simulink model "RRpendulum_digtwin_BLDC"  (R2024b)
settings: Solver=FixedStepAuto  StartTime=0.0  StopTime=inf  FixedStep=0.001  RelTol=1e-3  EnableMultiTasking=on
PreLoadFcn:
  | %define mechanical pars, init conditions
  | run RRpendulum_kinctrl_numericalsetup.mlx
  | 
  | %% parameters moved to model workspace
  | % sample time
  | %T_SAMPLE = 0.001;
  | 
  | %microsteps per turn of 200 step motor @ x16 microstepping
  | %STEPS_PER_TURN = 3200;
  | 
  | %encoder counts per turn
  | %COUNTS_PER_TURN = 2400;
model workspace (MAT data in the model file):
  COUNTS_PER_TURN_MOT = 8192
  COUNTS_PER_TURN_PEND = 2400
  MOTOR_VEL_RESOLUTION_DIV = 4
  PEND_VEL_RESOLUTION_DIV = 1
  T_SAMPLE = 0.001
undefined symbols (not defined in the file): b1_num, b2_num, dspblkCoreblockFVToolHelper, g_num, gcbh, l_num, m_num, q1_0, q2_0, r_num, satlimits, T01_num0, T12_num0, v1_0, v2_0, X, Y, Z
libraries: sm_lib x12, nesl_utility x7, simulink x2, fl_lib x2, ee_lib x2, raspberrypiCommlib x1
(part 2 of 2)

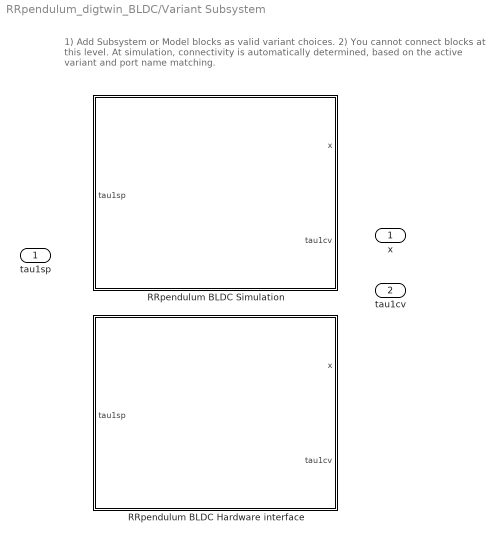
== system RRpendulum_digtwin_BLDC/Variant Subsystem ==
  note: 1) Add Subsystem or Model blocks as valid variant choices.
      | 2) You cannot connect blocks at this level. At simulation, connectivity is automatically
      | determined, based on the active variant and port name matching.
  tau1sp : Inport
  RRpendulum BLDC Hardware interface : Subsystem  VariantControl=(codegen)  mask{t_sample=T_SAMPLE, enc_cpt=COUNTS_PER_TURN_PEND, mot_cpt=COUNTS_PER_TURN_MOT, Nv2filt=10}
      mask prompts: t_sample "Sample time (s)"; enc_cpt "Pendulum Encoder CPT (x4)"; mot_cpt "Motor Encoder CPT (x4)"; Nv2filt "Moving average filter"
      mask Display:
      | image('pendulum_down_physical.PNG');
      | port_label('input', 1, 'tau1sp');
      | port_label('output', 1, 'x');
      | port_label('output', 2, 'tau1cv');
  RRpendulum BLDC Simulation : Subsystem  VariantControl=(sim)  mask{initstate=[q1_0; v1_0 ;q2_0; v2_0], satlimits=satlimits, g=g_num, m=m_num, r=r_num, l=l_num, b=[b1_num b2_num]}
      mask prompts: initstate "Initial state: [q1; v1; q2; v2]"; satlimits "Saturation limits axis 1: [vdot1max;v1max]"; g "Gravity: g"; m "Mass: m"; r "Radius: r"; l "Length: l"; b "Viscous damping factors: [b1;b2]"
      mask DialogControl MechanismGroupVar Prompt: Mechanism
      mask Display:
      | image('pendulum_down_simulation.PNG');
      | port_label('input', 1, 'tau1sp');
      | port_label('output', 1, 'x');
      | port_label('output', 2, 'tau1cv');
  x : Outport
  tau1cv : Outport  Port=2

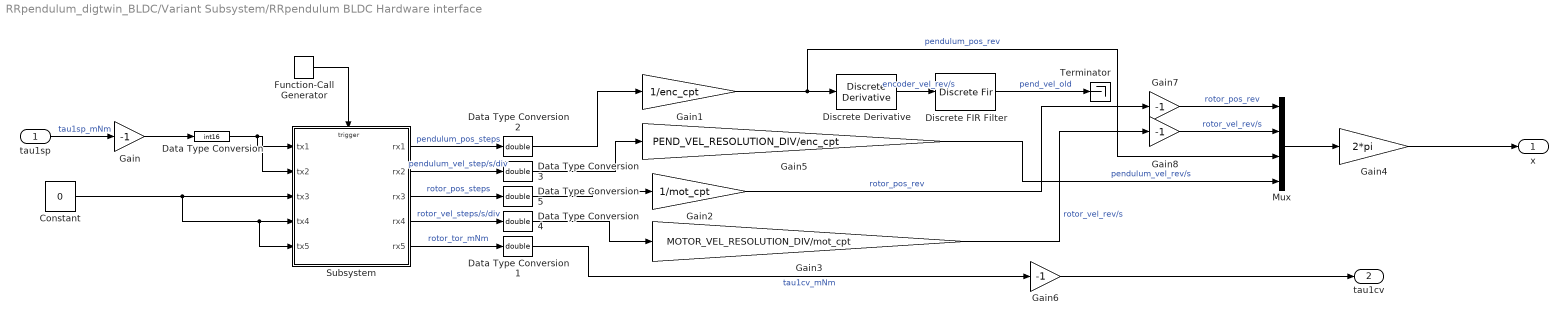
== system RRpendulum_digtwin_BLDC/Variant Subsystem/RRpendulum BLDC Hardware interface ==
  tau1sp : Inport
  Constant : Constant  Value=0  OutDataTypeStr=int16
  Data Type Conversion : DataTypeConversion  OutDataTypeStr=int16  SaturateOnIntegerOverflow=off  RndMeth=Floor
  Data Type Conversion{1..5} (5 alike) : DataTypeConversion  OutDataTypeStr=double  SaturateOnIntegerOverflow=off  RndMeth=Floor
  Discrete Derivative : simulink/Discrete/Discrete Derivative  gainval=1.0  ICPrevScaledInput=0.0  OutMin=[]  OutMax=[]  OutDataType=fixdt(1, 16)  OutScaling=2^-10  DoSatur=off
  Discrete FIR Filter : DiscreteFir  LoadFcn=dspblkCoreblockFVToolHelper(gcbh,'load');  Coefficients=ones(1,Nv2filt)/Nv2filt
      settings: CopyFcn=dspblkCoreblockFVToolHelper(gcbh,'copy');  DeleteFcn=dspblkCoreblockFVToolHelper(gcbh,'close');  ModelCloseFcn=dspblkCoreblockFVToolHelper(gcbh,'close');  PreSaveFcn=dspblkCoreblockFVToolHelper(gcbh,'presave');  PostSaveFcn=dspblkCoreblockFVToolHelper(gcbh,'postsave');  CloseFcn=dspblkCoreblockFVToolHelper(gcbh,'close');
  Function-Call Generator : simulink/Ports & Subsystems/Function-Call Generator  sample_time=t_sample  numberOfIterations=1  DisallowWideOutput=off
  Gain{,6..8} (4 alike) : Gain  Gain=-1
  Gain1 : Gain  Gain=1/enc_cpt
  Gain2 : Gain  Gain=1/mot_cpt
  Gain3 : Gain  Gain=MOTOR_VEL_RESOLUTION_DIV/mot_cpt
  Gain4 : Gain  Gain=2*pi
  Gain5 : Gain  Gain=PEND_VEL_RESOLUTION_DIV/enc_cpt
  Mux : Mux
  Subsystem : Subsystem
  Terminator : Terminator
  x : Outport
  tau1cv : Outport  Port=2
  wires:
  Data Type Conversion2/1 -> Gain1/1
  Data Type Conversion/1 -> Subsystem/2(tx2), Subsystem/1(tx1)
  Gain1/1 -> Discrete Derivative/1, Mux/3  "pendulum_pos_rev"
  Data Type Conversion3/1 -> Gain5/1
  Subsystem/1(rx1) -> Data Type Conversion2/1  "pendulum_pos_steps"
  Function-Call Generator/1 -> Subsystem/Trigger
  Subsystem/2(rx2) -> Data Type Conversion3/1  "pendulum_vel_step/s/div"
  Subsystem/4(rx4) -> Data Type Conversion4/1  "rotor_vel_steps/s/div"
  Gain3/1 -> Gain8/1  "rotor_vel_rev/s"
  Constant/1 -> Subsystem/5(tx5), Subsystem/4(tx4), Subsystem/3(tx3)
  Data Type Conversion4/1 -> Gain3/1
  tau1sp/1 -> Gain/1  "tau1sp_mNm"
  Gain2/1 -> Gain7/1  "rotor_pos_rev"
  Discrete Derivative/1 -> Discrete FIR Filter/1  "encoder_vel_rev/s"
  Mux/1 -> Gain4/1
  Discrete FIR Filter/1 -> Terminator/1  "pend_vel_old"
  Subsystem/5(rx5) -> Data Type Conversion1/1  "rotor_tor_mNm"
  Gain4/1 -> x/1
  Data Type Conversion1/1 -> Gain6/1  "tau1cv_mNm"
  Gain5/1 -> Mux/4  "pendulum_vel_rev/s"
  Subsystem/3(rx3) -> Data Type Conversion5/1  "rotor_pos_steps"
  Data Type Conversion5/1 -> Gain2/1
  Gain/1 -> Data Type Conversion/1
  Gain6/1 -> tau1cv/1
  Gain7/1 -> Mux/1  "rotor_pos_rev"
  Gain8/1 -> Mux/2  "rotor_vel_rev/s"

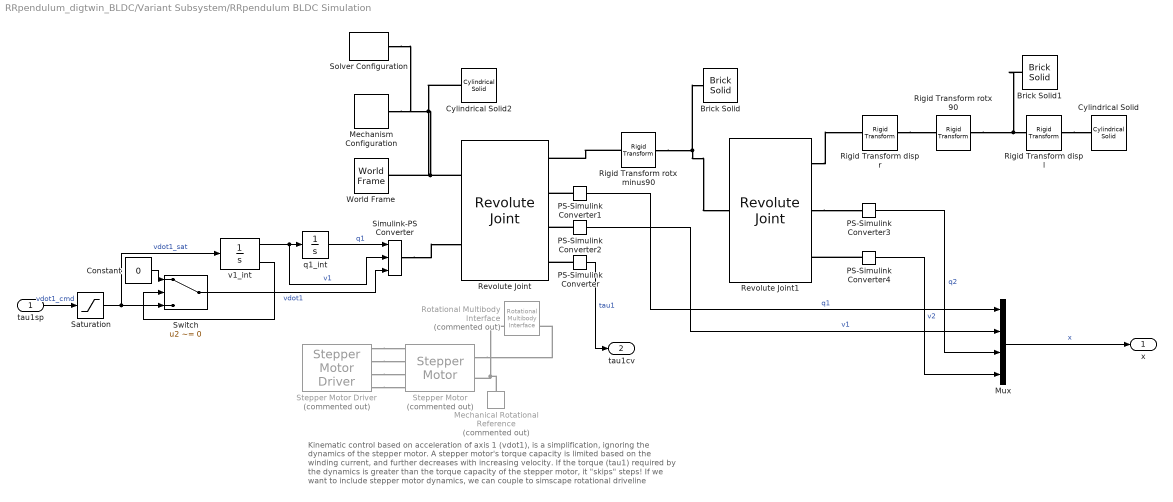
== system RRpendulum_digtwin_BLDC/Variant Subsystem/RRpendulum BLDC Simulation ==
  note: Kinematic control based on acceleration of axis 1 (vdot1), is a simplification, ignoring the dynamics of the stepper motor.
      |
      | A stepper motor's torque capacity is limited based on the winding current, and further decreases with increasing velocity. If the torque (tau1) required by the dynamics is greater than the torque capacity of the stepper motor, it "skips" steps!
      |
      | If we want to include stepper motor dynamics, we can couple to simscape rotational driveline
  tau1sp : Inport
  Brick Solid : sm_lib/Body Elements/Brick Solid  BrickDimensions=[0.001 0.001 r_num]  BrickDimensionsUnits=m  ExportEntireGeometry=off  InertiaType=CalculateFromGeometry  BasedOnType=Mass  Density=1000  DensityUnits=kg/m^3  Mass=0  MassUnits=kg  CenterOfMass=[0 0 0]  CenterOfMassUnits=m  MomentsOfInertia=[1 1 1]  MomentsOfInertiaUnits=kg*m^2  ProductsOfInertia=[0 0 0]  ProductsOfInertiaUnits=kg*m^2  GraphicType=FromGeometry  MarkerShape=Sphere  MarkerSize=10  GraphicVisPropType=SimpleVisualProperties  GraphicDiffuseColor=[0.5 0.5 0.5]  GraphicOpacity=1  GraphicSpecularColor=[0.5 0.5 0.5 1.0]  GraphicAmbientColor=[0.15 0.15 0.15 1.0]  GraphicEmissiveColor=[0.0 0.0 0.0 1.0]  GraphicShininess=75  DoExposeReferenceFrame=on  SerializedFrames=<Frames><Frame><Id>Frame1</Id><Value><Name>F1</Name><Origin><Source>GeometricFeature</Source><FeatureName>-z surface</FeatureName></Origin><PrimaryAxis><DefinedDirection>-Z</DefinedDirection><Source>GeometricFeature</Source><SourceDirection>+Z</SourceDirection><FeatureName>-z surface</FeatureName></PrimaryAxis><SecondaryAxis><DefinedDirection>+X</DefinedDirection><Source>ReferenceFrame</Source><SourceDirection>+X</SourceDirection><FeatureName></FeatureName></SecondaryAxis></Value></Frame></Frames>
  Brick Solid1 : sm_lib/Body Elements/Brick Solid  BrickDimensions=[0.001 0.001 l_num]  BrickDimensionsUnits=m  ExportEntireGeometry=off  InertiaType=CalculateFromGeometry  BasedOnType=Mass  Density=1000  DensityUnits=kg/m^3  Mass=0  MassUnits=kg  CenterOfMass=[0 0 0]  CenterOfMassUnits=m  MomentsOfInertia=[1 1 1]  MomentsOfInertiaUnits=kg*m^2  ProductsOfInertia=[0 0 0]  ProductsOfInertiaUnits=kg*m^2  GraphicType=FromGeometry  MarkerShape=Sphere  MarkerSize=10  GraphicVisPropType=SimpleVisualProperties  GraphicDiffuseColor=[0.5 0.5 0.5]  GraphicOpacity=1  GraphicSpecularColor=[0.5 0.5 0.5 1.0]  GraphicAmbientColor=[0.15 0.15 0.15 1.0]  GraphicEmissiveColor=[0.0 0.0 0.0 1.0]  GraphicShininess=75  DoExposeReferenceFrame=on  SerializedFrames=<Frames><Frame><Id>Frame1</Id><Value><Name>F1</Name><Origin><Source>GeometricFeature</Source><FeatureName>-z surface</FeatureName></Origin><PrimaryAxis><DefinedDirection>+Z</DefinedDirection><Source>GeometricFeature</Source><SourceDirection>+Z</SourceDirection><FeatureName>-z surface</FeatureName></PrimaryAxis><SecondaryAxis><DefinedDirection>+X</DefinedDirection><Source>ReferenceFrame</Source><SourceDirection>+X</SourceDirection><FeatureName></FeatureName></SecondaryAxis></Value></Frame></Frames>
  Constant : Constant  Value=0
  Cylindrical Solid : sm_lib/Body Elements/Cylindrical Solid  CylinderRadius=5  CylinderRadiusUnits=mm  CylinderLength=30  CylinderLengthUnits=mm  ExportEntireGeometry=off  InertiaType=PointMass  BasedOnType=Mass  Density=1000  DensityUnits=kg/m^3  Mass=m  MassUnits=kg  CenterOfMass=[0 0 0]  CenterOfMassUnits=m  MomentsOfInertia=[1 1 1]  MomentsOfInertiaUnits=kg*m^2  ProductsOfInertia=[0 0 0]  ProductsOfInertiaUnits=kg*m^2  GraphicType=FromGeometry  MarkerShape=Sphere  MarkerSize=10  GraphicVisPropType=SimpleVisualProperties  GraphicDiffuseColor=[0.5 0.5 0.5]  GraphicOpacity=1  GraphicSpecularColor=[0.5 0.5 0.5 1.0]  GraphicAmbientColor=[0.15 0.15 0.15 1.0]  GraphicEmissiveColor=[0.0 0.0 0.0 1.0]  GraphicShininess=75  DoExposeReferenceFrame=on  SerializedFrames=<Frames/>
  Cylindrical Solid2 : sm_lib/Body Elements/Cylindrical Solid  CylinderRadius=0.1*r_num  CylinderRadiusUnits=m  CylinderLength=l_num*1.25  CylinderLengthUnits=m  ExportEntireGeometry=off  InertiaType=CalculateFromGeometry  BasedOnType=Mass  Density=1000  DensityUnits=kg/m^3  Mass=0  MassUnits=kg  CenterOfMass=[0 0 0]  CenterOfMassUnits=m  MomentsOfInertia=[1 1 1]  MomentsOfInertiaUnits=kg*m^2  ProductsOfInertia=[0 0 0]  ProductsOfInertiaUnits=kg*m^2  GraphicType=FromGeometry  MarkerShape=Sphere  MarkerSize=10  GraphicVisPropType=SimpleVisualProperties  GraphicDiffuseColor=[0.5 0.5 0.5]  GraphicOpacity=1  GraphicSpecularColor=[0.5 0.5 0.5 1.0]  GraphicAmbientColor=[0.15 0.15 0.15 1.0]  GraphicEmissiveColor=[0.0 0.0 0.0 1.0]  GraphicShininess=75  DoExposeReferenceFrame=on  SerializedFrames=<Frames><Frame><Id>Frame1</Id><Value><Name>F1</Name><Origin><Source>GeometricFeature</Source><FeatureName>top surface</FeatureName></Origin><PrimaryAxis><DefinedDirection>+Z</DefinedDirection><Source>ReferenceFrame</Source><SourceDirection>+Z</SourceDirection><FeatureName></FeatureName></PrimaryAxis><SecondaryAxis><DefinedDirection>+X</DefinedDirection><Source>ReferenceFrame</Source><SourceDirection>+X</SourceDirection><FeatureName></FeatureName></SecondaryAxis></Value></Frame></Frames>
  Mechanical Rotational Reference : fl_lib/Mechanical/Rotational Elements/Mechanical Rotational Reference  Commented=on
  Mechanism Configuration : sm_lib/Utilities/Mechanism Configuration  UniformGravity=Constant  GravityVector=[0 0 -g]  GravityVectorUnits=m/s^2  LinearizationDelta=0.001  JointModeTransitionNonlinearIterations=2
  Mux : Mux
  PS-Simulink Converter : nesl_utility/PS-Simulink Converter  PhysicalDomain=network_engine_domain  SubClassName=ps_output  LeftPortType=input  RightPortType=output  PseudoPeriodic=off  Frequencies=[]  VectorFormat=inherit  Unit=N*m  AffineConversion=off
  PS-Simulink Converter1 : nesl_utility/PS-Simulink Converter  PhysicalDomain=network_engine_domain  SubClassName=ps_output  LeftPortType=input  RightPortType=output  PseudoPeriodic=off  Frequencies=[]  VectorFormat=inherit  Unit=rad  AffineConversion=off
  PS-Simulink Converter2 : nesl_utility/PS-Simulink Converter  PhysicalDomain=network_engine_domain  SubClassName=ps_output  LeftPortType=input  RightPortType=output  PseudoPeriodic=off  Frequencies=[]  VectorFormat=inherit  Unit=rad/s  AffineConversion=off
  PS-Simulink Converter3 : nesl_utility/PS-Simulink Converter  PhysicalDomain=network_engine_domain  SubClassName=ps_output  LeftPortType=input  RightPortType=output  PseudoPeriodic=off  Frequencies=[]  VectorFormat=inherit  Unit=rad  AffineConversion=off
  PS-Simulink Converter4 : nesl_utility/PS-Simulink Converter  PhysicalDomain=network_engine_domain  SubClassName=ps_output  LeftPortType=input  RightPortType=output  PseudoPeriodic=off  Frequencies=[]  VectorFormat=inherit  Unit=rad/s  AffineConversion=off
  Revolute Joint : sm_lib/Joints/Revolute Joint  JointMode=Normal  CompositeWrenchDir=FollowerOnBase  CompositeWrenchFrame=BaseFrame  SenseConstraintForce=off  SenseConstraintTorque=off  SenseTotalForce=off  SenseTotalTorque=off  PositionTargetSpecify=on  PositionTargetPriority=High  PositionTargetValue=initstate(1)  PositionTargetValueUnits=rad  VelocityTargetSpecify=on  VelocityTargetPriority=High  VelocityTargetValue=initstate(2)  VelocityTargetValueUnits=rad/s  EquilibriumPosition=0  EquilibriumPositionUnits=deg  SpringStiffness=0  SpringStiffnessUnits=N*m/deg  DampingCoefficient=b(1)  DampingCoefficientUnits=N*m*s/rad  LowerLimitSpecify=off  LowerLimitBound=-90  LowerLimitBoundUnits=deg  LowerLimitStiffness=1e4  LowerLimitStiffnessUnits=N*m/deg  LowerLimitDamping=10  LowerLimitDampingUnits=N*m/(deg/s)  LowerLimitTransitionRegionWidth=0.1  LowerLimitTransitionRegionWidthUnits=deg  UpperLimitSpecify=off  UpperLimitBound=90  UpperLimitBoundUnits=deg  UpperLimitStiffness=1e4  UpperLimitStiffnessUnits=N*m/deg  UpperLimitDamping=10  UpperLimitDampingUnits=N*m/(deg/s)  UpperLimitTransitionRegionWidth=0.1  UpperLimitTransitionRegionWidthUnits=deg  TorqueActuationMode=ComputedTorque  MotionActuationMode=InputMotion  SensePosition=on  SenseVelocity=on  SenseAcceleration=off  SenseTorqueForce=on  SenseLowerLimitTorqueForce=off  SenseUpperLimitTorqueForce=off
  Revolute Joint1 : sm_lib/Joints/Revolute Joint  JointMode=Normal  CompositeWrenchDir=FollowerOnBase  CompositeWrenchFrame=BaseFrame  SenseConstraintForce=off  SenseConstraintTorque=off  SenseTotalForce=off  SenseTotalTorque=off  PositionTargetSpecify=on  PositionTargetPriority=High  PositionTargetValue=initstate(3)  PositionTargetValueUnits=rad  VelocityTargetSpecify=on  VelocityTargetPriority=High  VelocityTargetValue=initstate(4)  VelocityTargetValueUnits=rad/s  EquilibriumPosition=0  EquilibriumPositionUnits=deg  SpringStiffness=0  SpringStiffnessUnits=N*m/deg  DampingCoefficient=b(2)  DampingCoefficientUnits=N*m*s/rad  LowerLimitSpecify=off  LowerLimitBound=-90  LowerLimitBoundUnits=deg  LowerLimitStiffness=1e4  LowerLimitStiffnessUnits=N*m/deg  LowerLimitDamping=10  LowerLimitDampingUnits=N*m/(deg/s)  LowerLimitTransitionRegionWidth=0.1  LowerLimitTransitionRegionWidthUnits=deg  UpperLimitSpecify=off  UpperLimitBound=90  UpperLimitBoundUnits=deg  UpperLimitStiffness=1e4  UpperLimitStiffnessUnits=N*m/deg  UpperLimitDamping=10  UpperLimitDampingUnits=N*m/(deg/s)  UpperLimitTransitionRegionWidth=0.1  UpperLimitTransitionRegionWidthUnits=deg  TorqueActuationMode=NoTorque  MotionActuationMode=ComputedMotion  SensePosition=on  SenseVelocity=on  SenseAcceleration=off  SenseTorqueForce=off  SenseLowerLimitTorqueForce=off  SenseUpperLimitTorqueForce=off
  Rigid Transform disp l : sm_lib/Frames and Transforms/Rigid Transform  RotationMethod=None  FollAlignAxisA=+X  BaseAlignAxisA=+Y  FollAlignAxisB=+Y  BaseAlignAxisB=+Z  RotationStandardAxis=+Z  RotationAngle=0  RotationAngleUnits=deg  RotationArbitraryAxis=[0 0 1]  RotationSequenceAxes=FollowerAxes  RotationSequence=XYX  RotationSequenceAngles=[0 0 0]  RotationSequenceAnglesUnits=deg  RotationMatrix=rotx(90)  Quaternion=[1 0 0 0]  TranslationMethod=StandardAxis  TranslationCartesianOffset=T12_num0(1:3,4)'  TranslationCartesianOffsetUnits=m  TranslationStandardAxis=-Z  TranslationStandardOffset=l  TranslationStandardOffsetUnits=m  TranslationROffset=0  TranslationROffsetUnits=m  TranslationThetaOffset=0  TranslationThetaOffsetUnits=deg  TranslationZOffset=0  TranslationZOffsetUnits=m
  Rigid Transform disp r : sm_lib/Frames and Transforms/Rigid Transform  RotationMethod=None  FollAlignAxisA=+X  BaseAlignAxisA=+Y  FollAlignAxisB=+Y  BaseAlignAxisB=+Z  RotationStandardAxis=+Z  RotationAngle=0  RotationAngleUnits=deg  RotationArbitraryAxis=[0 0 1]  RotationSequenceAxes=FollowerAxes  RotationSequence=XYX  RotationSequenceAngles=[0 0 0]  RotationSequenceAnglesUnits=deg  RotationMatrix=T12_num0(1:3,1:3)  Quaternion=[1 0 0 0]  TranslationMethod=StandardAxis  TranslationCartesianOffset=T12_num0(1:3,4)'  TranslationCartesianOffsetUnits=m  TranslationStandardAxis=+Z  TranslationStandardOffset=r  TranslationStandardOffsetUnits=m  TranslationROffset=0  TranslationROffsetUnits=m  TranslationThetaOffset=0  TranslationThetaOffsetUnits=deg  TranslationZOffset=0  TranslationZOffsetUnits=m
  Rigid Transform rotx 90 : sm_lib/Frames and Transforms/Rigid Transform  RotationMethod=RotationMatrix  FollAlignAxisA=+X  BaseAlignAxisA=+Y  FollAlignAxisB=+Y  BaseAlignAxisB=+Z  RotationStandardAxis=+Z  RotationAngle=0  RotationAngleUnits=deg  RotationArbitraryAxis=[0 0 1]  RotationSequenceAxes=FollowerAxes  RotationSequence=XYX  RotationSequenceAngles=[0 0 0]  RotationSequenceAnglesUnits=deg  RotationMatrix=rotx(90)  Quaternion=[1 0 0 0]  TranslationMethod=None  TranslationCartesianOffset=T12_num0(1:3,4)'  TranslationCartesianOffsetUnits=m  TranslationStandardAxis=+Z  TranslationStandardOffset=0  TranslationStandardOffsetUnits=m  TranslationROffset=0  TranslationROffsetUnits=m  TranslationThetaOffset=0  TranslationThetaOffsetUnits=deg  TranslationZOffset=0  TranslationZOffsetUnits=m
  Rigid Transform rotx minus90 : sm_lib/Frames and Transforms/Rigid Transform  RotationMethod=RotationMatrix  FollAlignAxisA=+X  BaseAlignAxisA=+Y  FollAlignAxisB=+Y  BaseAlignAxisB=+Z  RotationStandardAxis=+Z  RotationAngle=0  RotationAngleUnits=deg  RotationArbitraryAxis=[0 0 1]  RotationSequenceAxes=FollowerAxes  RotationSequence=XYX  RotationSequenceAngles=[0 0 0]  RotationSequenceAnglesUnits=deg  RotationMatrix=rotx(-90)  Quaternion=[1 0 0 0]  TranslationMethod=None  TranslationCartesianOffset=T01_num0(1:3,4)'  TranslationCartesianOffsetUnits=m  TranslationStandardAxis=+Z  TranslationStandardOffset=0  TranslationStandardOffsetUnits=m  TranslationROffset=0  TranslationROffsetUnits=m  TranslationThetaOffset=0  TranslationThetaOffsetUnits=deg  TranslationZOffset=0  TranslationZOffsetUnits=m
  Rotational Multibody Interface : fl_lib/Mechanical/Multibody Interfaces/Rotational Multibody Interface  Commented=on
  Saturation : Saturate  UpperLimit=satlimits(1)  LowerLimit=-satlimits(1)
  Simulink-PS Converter : nesl_utility/Simulink-PS Converter  PhysicalDomain=network_engine_domain  SubClassName=ps_input  LeftPortType=input  RightPortType=output  PseudoPeriodic=off  Frequencies=[]  NoiseDistribution=none  NoiseParameters=[]  Unit=rad  AffineConversion=off  FilteringAndDerivatives=provide  SimscapeFilterOrder=1  InputFilterTimeConstant=0.001  UdotUserProvided=2
  Solver Configuration : nesl_utility/Solver Configuration  PhysicalDomain=network_engine_domain  SubClassName=solver  LeftPortType=input  RightPortType=generic  Tones=[]  Harmonics=[]  SimulateNoise=off  Profile=off  UseLocalSampling=off  EnableSwitchedLinearOptims=on  FrequencyDomain=off  UseCCode=off  RelTol=0.001  AbsTol=0.001  MinStep=1e-09  ToWorkspace=off  RevertToSquareIcSolve=off  NumHomotopyIterations=100  PhasorMode=off  PhasorModeNumHarmonics=1  ConsistencySolver=NEWTON_XTOL_AFTER_FTOL  IndexReductionMethod=DerivativeReplacement  DoDC=off  ResidualTolerance=1e-09  ConsistencyTolSource=GLOBAL  ConsistencyAbsTol=0.001  ConsistencyRelTol=0.001  ConsistencyTolFactor=0.0001  UseLocalSolver=off  LocalSolverChoice=NE_BACKWARD_EULER_ADVANCER  ResolveIndetEquations=on  FunctionEvalNumThread=1  LocalSolverSampleTime=0.001  DoFixedCost=off  MaxNonlinIter=3  MaxModeIter=2  ComputeImpulses=off  ImpulseIterations=2  LinearAlgebra=auto  LinearAlgebraNumThread=0  EquationFormulation=NE_TIME_EF  DelaysMemoryBudget=1024  AutomaticFiltering=on  FilteringTimeConstant=0.001  PartitionStorageMethod=AS_NEEDED  PartitionMemoryBudget=1024  PartitionMethod=ROBUST  MultibodyUseLocalSolver=off  MultibodyLocalSolverChoice=ODE1  MultibodyLocalSolverSampleTime=0.001
  Stepper Motor : ee_lib/Electromechanical/Reluctance & Stepper/Stepper Motor  Commented=on  step_or_av=ee.enum.electromech.simulationMode.stepping  Ra=0.55 Ohm  La=1.5e-3 H  Km=0.19 N*m/A  Td=0 N*m  Rm=inf Ohm  w_vec=[0, 1000, 3000] rpm  T_vec=[2, 2, 1] N*m  assert_if_slipping=ee.enum.assertAction.none  J_total=1e-4 kg*m^2  max_step_rate=10 Hz  Step=1.8 deg  J=4.5e-5 kg*m^2  B=8.0e-4 N*m*s/rad  speed0=0 rpm  theta0=0 deg  alpha=[.00393, .00393] 1/K  Tmeas=25 degC  Tmeas2=125 degC  T_vec2=[1.7, 1.7, .85] N*m  half_stepping=ee.enum.electromech.steppingModeAveraged.fullStep  thermal_masses=[100, 100] J/K  initial_temperatures=[25, 25] degC  rotor_thermal_mass=50 J/K  rotor_initial_temperature=25 degC  Rm_percent_rotor=90
      settings: InternalSimscapePortConfiguration="{\"Bottom\":[],\"Left\":[{\"id\":\"pA\",\"label\":\"A+\",\"type\":\"foundation.electrical.electrical\"},{\"id\":\"nA\",\"label\":\"A-\",\"type\":\"foundation.electrical.electrical\"},{\"id\":\"pB\",\"label\":\"B+\",\"type\":\"foundation.electrical.electrical\"},{\"id\":\"nB\",\"label\":\"B-\",\"type\":\"foundation.electrical.electrical\"}],\"Right\":[{\"id\":\"R\",\"label\":\"R\",\"type\":\"foundation.mechanical.rotational.rotational\"},{\"id\":\"C\",\"label\":\"C\",\"type\":\"foundation.mechanical.rotational.rotational\"}],\"Top\":[]}"
  Stepper Motor Driver : ee_lib/Electromechanical/Reluctance & Stepper/Stepper Motor Driver  Commented=on  step_or_av=ee.enum.electromech.simulationMode.stepping  step_rate_per_volt=10 Hz/V  Venable=2.5 V  Vreverse=2.5 V  supply_ports=ee.enum.supply_ports.hidesupply  Vm=10 V  Vsupply=10 V  half_stepping=ee.enum.electromech.steppingModeAveraged.fullStep  stepping_mode=ee.enum.electromech.steppingMode.fullStep  numMicroSteps=4  Im=1.2 A
      settings: InternalSimscapePortConfiguration="{\"Bottom\":[],\"Left\":[{\"id\":\"ENA\",\"label\":\"ENA\",\"type\":\"foundation.electrical.electrical\"},{\"id\":\"REF\",\"label\":\"REF\",\"type\":\"foundation.electrical.electrical\"},{\"id\":\"REV\",\"label\":\"REV\",\"type\":\"foundation.electrical.electrical\"}],\"Right\":[{\"id\":\"pA\",\"label\":\"A+\",\"type\":\"foundation.electrical.electrical\"},{\"id\":\"nA\",\"label\":\"A-\",\"type\":\"foundation.electrical.electrical\"},{\"id\":\"pB\",\"label\":\"B+\",\"type\":\"foundation.electrical.electrical\"},{\"id\":\"nB\",\"label\":\"B-\",\"type\":\"foundation.electrical.electrical\"}],\"Top\":[]}"
  Switch : Switch  Criteria=u2 ~= 0  SaturateOnIntegerOverflow=off  InputSameDT=off
  World Frame : sm_lib/Frames and Transforms/World Frame
  q1_int : Integrator  InitialCondition=initstate(1)  UpperSaturationLimit=satlimits(3)  LowerSaturationLimit=-satlimits(3)
  v1_int : Integrator  InitialCondition=initstate(2)  LimitOutput=on  UpperSaturationLimit=satlimits(2)  LowerSaturationLimit=-satlimits(2)  ShowSaturationPort=on
  x : Outport  PortDimensions=[4,1]
  tau1cv : Outport  Port=2
  wires:
  PS-Simulink Converter3/1 -> Mux/3  "q2"
  Mux/1 -> x/1  "x"
  tau1sp/1 -> Saturation/1  "vdot1_cmd"
  v1_int/1 -> Simulink-PS Converter/2, q1_int/1  "v1"
  PS-Simulink Converter4/1 -> Mux/4  "v2"
  q1_int/1 -> Simulink-PS Converter/1  "q1"
  PS-Simulink Converter1/1 -> Mux/1  "q1"
  PS-Simulink Converter2/1 -> Mux/2  "v1"
  v1_int/2 -> Switch/2
  Constant/1 -> Switch/1
  Saturation/1 -> v1_int/1, Switch/3  "vdot1_sat"
  Switch/1 -> Simulink-PS Converter/3  "vdot1"
  PS-Simulink Converter/1 -> tau1cv/1  "tau1"
  connections:
  Stepper Motor Driver/RConn2 -- Stepper Motor/LConn2
  Rotational Multibody Interface/LConn2 -- Mechanical Rotational Reference/LConn1 -- Stepper Motor/RConn2
  Revolute Joint/LConn1 -- Cylindrical Solid2/LConn1 -- Solver Configuration/RConn1 -- Mechanism Configuration/RConn1 -- World Frame/RConn1
  PS-Simulink Converter4/LConn1 -- Revolute Joint1/RConn3
  Rigid Transform rotx 90/RConn1 -- Brick Solid1/LConn1 -- Rigid Transform disp l/LConn1
  Simulink-PS Converter/RConn1 -- Revolute Joint/LConn2
  Revolute Joint1/RConn1 -- Rigid Transform disp r/LConn1
  Stepper Motor Driver/RConn3 -- Stepper Motor/LConn3
  Rigid Transform rotx minus90/RConn1 -- Revolute Joint1/LConn1 -- Brick Solid/LConn1
  Stepper Motor/RConn1 -- Rotational Multibody Interface/RConn2
  Rigid Transform disp l/RConn1 -- Cylindrical Solid/RConn1
  Rigid Transform rotx minus90/LConn1 -- Revolute Joint/RConn1
  Stepper Motor Driver/RConn1 -- Stepper Motor/LConn1
  Rigid Transform disp r/RConn1 -- Rigid Transform rotx 90/LConn1
  PS-Simulink Converter/LConn1 -- Revolute Joint/RConn4
  Revolute Joint1/RConn2 -- PS-Simulink Converter3/LConn1
  Stepper Motor Driver/RConn4 -- Stepper Motor/LConn4
  PS-Simulink Converter1/LConn1 -- Revolute Joint/RConn2
  PS-Simulink Converter2/LConn1 -- Revolute Joint/RConn3

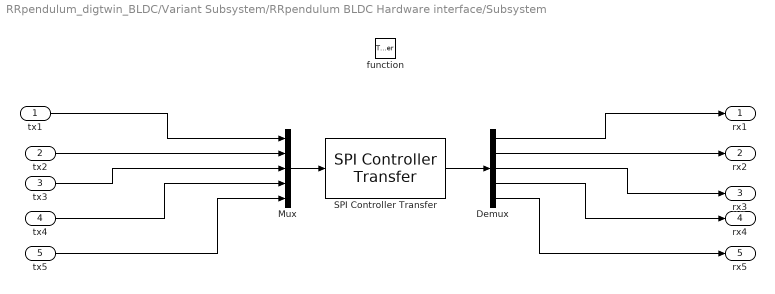
== system RRpendulum_digtwin_BLDC/Variant Subsystem/RRpendulum BLDC Hardware interface/Subsystem ==
  tx1 : Inport
  tx2 : Inport  Port=2
  tx3 : Inport  Port=3
  tx4 : Inport  Port=4
  tx5 : Inport  Port=5
  function : TriggerPort  TriggerType=function-call  VariantControl=(inherit)
  Demux : Demux  Outputs=5
  Mux : Mux  Inputs=5
  SPI Controller Transfer : raspberrypiCommlib/SPI Controller Transfer  BoardProperty=Pi 4 Model B  SSPin=SPI0_CE0  SPIModule=uint32(0)  Mode=Master  BusSpeed=1000000  Pin=uint32(0)  FirstBitToTransfer=Most significant bit (MSB)  ClockMode=0  BlockFunction=Transfer  RegisterAddress=0  OutputDataType=int8  OutputDataLength=1
  rx1 : Outport
  rx2 : Outport  Port=2
  rx3 : Outport  Port=3
  rx4 : Outport  Port=4
  rx5 : Outport  Port=5
  wires:
  SPI Controller Transfer/1 -> Demux/1
  tx1/1 -> Mux/1
  Demux/1 -> rx1/1
  tx2/1 -> Mux/2
  Mux/1 -> SPI Controller Transfer/1
  Demux/2 -> rx2/1
  tx3/1 -> Mux/3
  Demux/3 -> rx3/1
  tx4/1 -> Mux/4
  Demux/4 -> rx4/1
  tx5/1 -> Mux/5
  Demux/5 -> rx5/1

== stateflow chart RRpendulum_digtwin_BLDC/Controller ==
  settings: updateMethod=DISCRETE  sampleTime=T_SAMPLE
  state Startup
    % wait for measured torque to be NOT -999 (this means no init)
  state Startup1
    Torque_cmd = 0;
  state Swingup
  state Stabilize
    en:
    if (abs(pi-states(3)) < abs(-pi-states(3)))
    ref_state = [0;0;pi;0];
    else
    ref_state = [0;0;-pi;0];
    end
    en,du:
    Torque_cmd=K*(ref_state-states);
    %(gains to be determined, also consider adding fancy control routines to make pendulum dance)
  (default) -> Startup
  Startup -> Startup1
  Startup1 -> Swingup : after(.2,sec)
  Swingup -> Stabilize : [abs(abs(states(3))-pi)<epsilon]
  data: tau1cv input; Etot input; Ekin input; Epot input; Torque_cmd output double size=1; states input; K parameter; epsilon parameter; g_num parameter; m_num parameter; r_num parameter; l_num parameter; Etgt local; deadzone local; stiffness local; accelpulseampl local; accelpulsetime local; q2zcpos input; q2zcneg input; q2pkneg input; q2pkpos input; ref_state local

== matlab function RRpendulum_digtwin_BLDC/MATLAB Function ==
  data: Etot output; Ekin output; Epot output; states input; g_num parameter; m_num parameter; r_num parameter; l_num parameter
function [Etot,Ekin,Epot]=calc_energy(states, g_num, m_num, r_num, l_num)
%q1=states(1);
v1=states(2);
q2=states(3);
v2=states(4);

Ekin=l_num^2*m_num*(v1^2 + v2^2)/2 + m_num*r_num^2*v1^2/2 - l_num^2*m_num*cos(q2)^2*v1^2/2 + l_num*m_num*r_num*cos(q2)*v2*v1;
Epot = -g_num*l_num*m_num*cos(q2)+m_num*g_num*l_num;
Etot = Ekin+Epot;
